simulink model "stateSpace"  (R2023b)
settings: Solver=VariableStepAuto  StartTime=0.0  StopTime=10  RelTol=1e-3  EnableMultiTasking=on
values from neighbouring files (symbols this model uses):
  g = 9.80665    [RegulatorLiniarizare2.m]
  I_r_A = I_r_B + m_r*l_AB^2    (= 0.00169018666667)    [RegulatorLiniarizare2.m]
  I_w_A = I_w_C + m_w*l_AC^2    (= 0.001261425)    [RegulatorLiniarizare2.m]
  I_w_C = 0.5*m_w*R^2    (= 8.6875e-05)    [RegulatorLiniarizare2.m]
  l_AB = l/2    (= 0.065)    [RegulatorLiniarizare2.m]
  l_AC = l    (= 0.13)    [RegulatorLiniarizare2.m]
  m_r = 0.2948    [RegulatorLiniarizare2.m]
  m_w = 0.0695    [RegulatorLiniarizare2.m]
settings Model: Creator=bkhusain  LastModifiedBy=tudorn
settings SolverCC: AlgebraicLoopSolver=TrustRegion
settings DataIOCC: LimitDataPoints=on  MaxDataPoints=10000
settings OptimizationCC: ReuseModelBlockBuffer=off  LifeSpan=inf
settings DebuggingCC: UnconnectedInputMsg=warning  UnconnectedOutputMsg=warning  UnconnectedLineMsg=warning  AllowSymbolicDim=off  SFUnexpectedBacktrackingDiag=warning  SFNoUnconditionalDefaultTransitionDiag=warning  SFExecutionAtInitializationDiag=none  ArithmeticOperatorsInVariantConditions=warning
settings ModelReferenceCC: EnableRefExpFcnMdlSchedulingChecks=on
settings SFSimCC: SimUseLocalCustomCode=off  CustomCodeUndefinedFunction=UseInterfaceOnly
settings RTWCC: RTWUseLocalCustomCode=off
settings CodeAppCC: StateflowObjectComments=on
settings GRTTargetCC: TargetLangStandard=C89/C90 (ANSI)
settings ConfigComp: CovMetricSettings=dw  CovSaveCumulativeToWorkspaceVar=on  CovSaveSingleToWorkspaceVar=on  CovExternalEMLEnable=off  CovSFcnEnable=off
settings SimscapeCC: SimscapeLogType=all  SimscapeLogSimulationStatistics=on  SimscapeLogDataHistory=10000

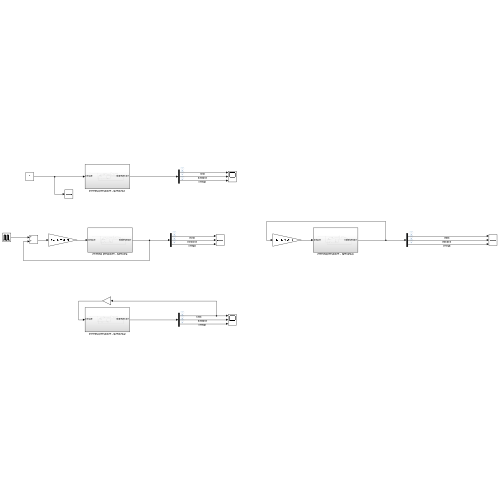
[thumbnail: Simulink's stored preview of the top-level diagram]
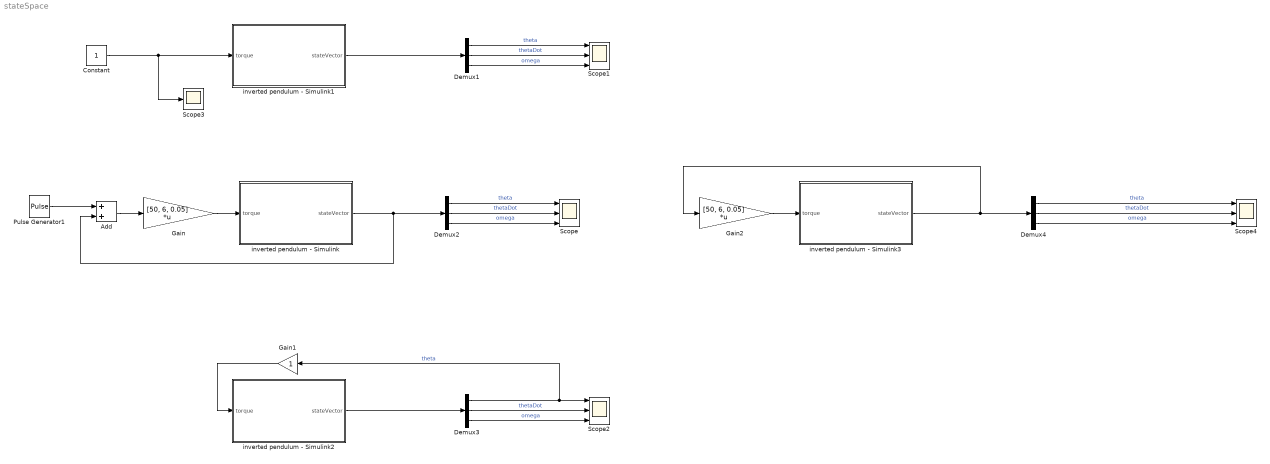
== system stateSpace ==
  Add : Sum
  Constant : Constant
  Demux{1..4} (4 alike) : Demux  Outputs=3
  Gain : Gain  Gain="[50,  6,  0.05]"  Multiplication=Matrix(K*u)
  Gain1 : Gain
  Gain2 : Gain  Gain="[50,  6,  0.05]"  Multiplication=Matrix(K*u)
  Pulse Generator1 : DiscretePulseGenerator  PulseType=Time based  Amplitude=0.5  Period=5  PulseWidth=5
  Scope{,1..2,4} (4 alike) : Scope  NumInputPorts=3
  Scope3 : Scope
  inverted pendulum - Simulink : Subsystem
  inverted pendulum - Simulink1 : Subsystem
  inverted pendulum - Simulink2 : Subsystem
  inverted pendulum - Simulink3 : Subsystem
  wires:
  Demux2/1 -> Scope/1  "theta"
  Demux2/3 -> Scope/3  "omega"
  Demux2/2 -> Scope/2  "thetaDot"
  Gain/1 -> inverted pendulum - Simulink/1(torque)
  Demux1/2 -> Scope1/2  "thetaDot"
  Demux1/3 -> Scope1/3  "omega"
  inverted pendulum - Simulink1/1(stateVector) -> Demux1/1
  Demux1/1 -> Scope1/1  "theta"
  Constant/1 -> Scope3/1, inverted pendulum - Simulink1/1(torque)
  Demux3/2 -> Scope2/2  "thetaDot"
  inverted pendulum - Simulink2/1(stateVector) -> Demux3/1
  Demux3/3 -> Scope2/3  "omega"
  Demux3/1 -> Gain1/1, Scope2/1  "theta"
  Gain1/1 -> inverted pendulum - Simulink2/1(torque)
  Add/1 -> Gain/1
  Pulse Generator1/1 -> Add/1
  inverted pendulum - Simulink/1(stateVector) -> Add/2, Demux2/1
  inverted pendulum - Simulink3/1(stateVector) -> Gain2/1, Demux4/1
  Gain2/1 -> inverted pendulum - Simulink3/1(torque)
  Demux4/2 -> Scope4/2  "thetaDot"
  Demux4/1 -> Scope4/1  "theta"
  Demux4/3 -> Scope4/3  "omega"

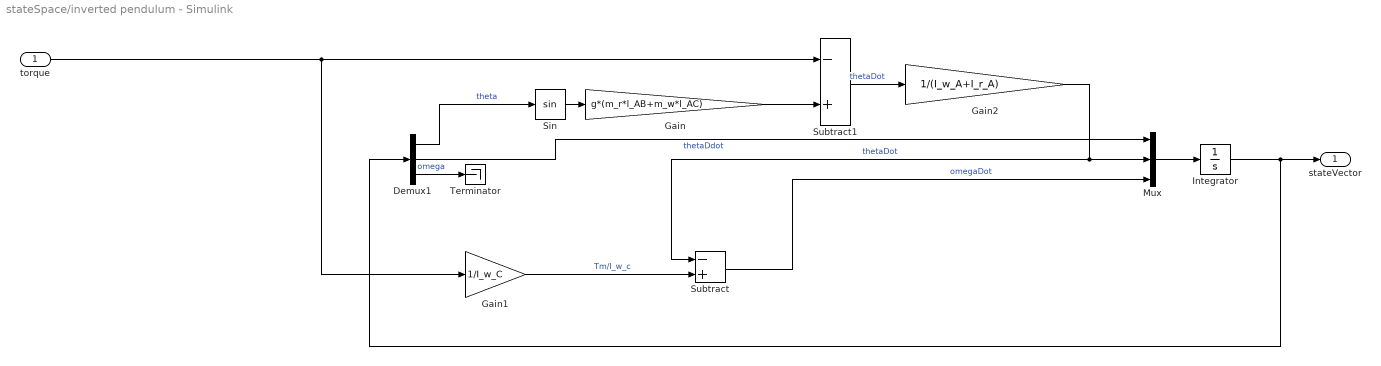
== system stateSpace/inverted pendulum - Simulink ==
  torque : Inport
  Demux1 : Demux  Outputs=3
  Gain : Gain  Gain=g*(m_r*l_AB+m_w*l_AC)
  Gain1 : Gain  Gain=1/I_w_C
  Gain2 : Gain  Gain=1/(I_w_A+I_r_A)
  Integrator : Integrator  InitialCondition=[60*pi/180, 0,0]
  Mux : Mux  Inputs=3
  Sin : Trigonometry
  Subtract : Sum  Inputs=-+
  Subtract1 : Sum  Inputs=-+
  Terminator : Terminator
  stateVector : Outport
  wires:
  Demux1/3 -> Terminator/1  "omega"
  Gain1/1 -> Subtract/2  "Tm/I_w_c"
  Demux1/1 -> Sin/1  "theta"
  Gain2/1 -> Subtract/1, Mux/2  "thetaDot"
  Gain/1 -> Subtract1/2
  Subtract1/1 -> Gain2/1  "thetaDot"
  Subtract/1 -> Mux/3  "omegaDot"
  Demux1/2 -> Mux/1  "thetaDdot"
  torque/1 -> Subtract1/1, Gain1/1
  Sin/1 -> Gain/1
  Integrator/1 -> stateVector/1, Demux1/1
  Mux/1 -> Integrator/1

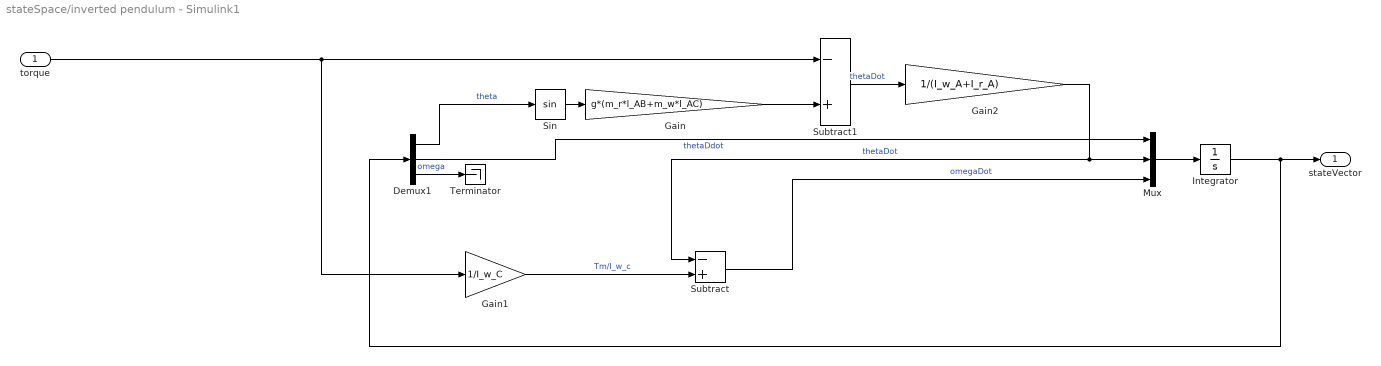
== system stateSpace/inverted pendulum - Simulink1 ==
  torque : Inport
  Demux1 : Demux  Outputs=3
  Gain : Gain  Gain=g*(m_r*l_AB+m_w*l_AC)
  Gain1 : Gain  Gain=1/I_w_C
  Gain2 : Gain  Gain=1/(I_w_A+I_r_A)
  Integrator : Integrator  InitialCondition=[30*pi/180, 0,0]
  Mux : Mux  Inputs=3
  Sin : Trigonometry
  Subtract : Sum  Inputs=-+
  Subtract1 : Sum  Inputs=-+
  Terminator : Terminator
  stateVector : Outport
  wires:
  Demux1/3 -> Terminator/1  "omega"
  Gain1/1 -> Subtract/2  "Tm/I_w_c"
  Demux1/1 -> Sin/1  "theta"
  Gain2/1 -> Subtract/1, Mux/2  "thetaDot"
  Gain/1 -> Subtract1/2
  Subtract1/1 -> Gain2/1  "thetaDot"
  Subtract/1 -> Mux/3  "omegaDot"
  Demux1/2 -> Mux/1  "thetaDdot"
  torque/1 -> Subtract1/1, Gain1/1
  Sin/1 -> Gain/1
  Integrator/1 -> stateVector/1, Demux1/1
  Mux/1 -> Integrator/1

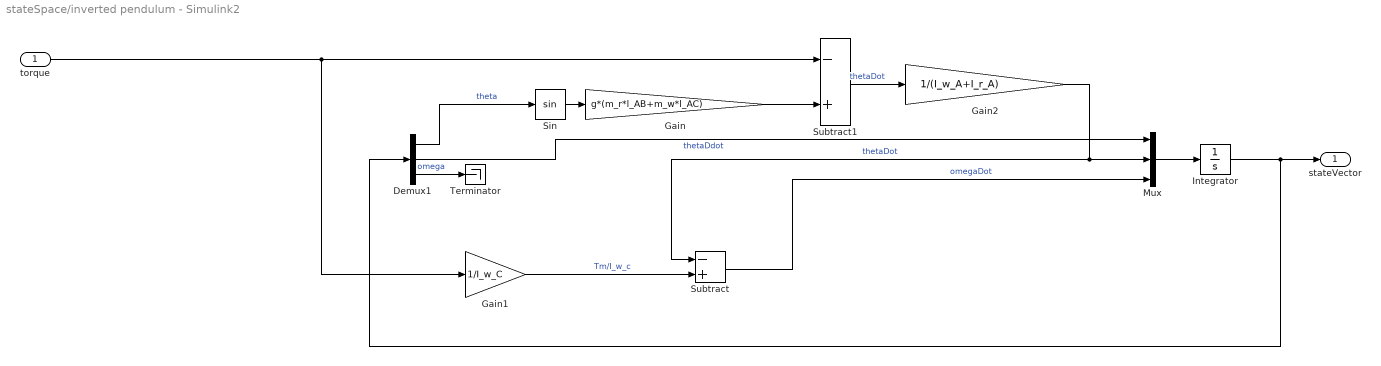
== system stateSpace/inverted pendulum - Simulink2 ==
  torque : Inport
  Demux1 : Demux  Outputs=3
  Gain : Gain  Gain=g*(m_r*l_AB+m_w*l_AC)
  Gain1 : Gain  Gain=1/I_w_C
  Gain2 : Gain  Gain=1/(I_w_A+I_r_A)
  Integrator : Integrator  InitialCondition=[60*pi/180, 0,0]
  Mux : Mux  Inputs=3
  Sin : Trigonometry
  Subtract : Sum  Inputs=-+
  Subtract1 : Sum  Inputs=-+
  Terminator : Terminator
  stateVector : Outport
  wires:
  Demux1/3 -> Terminator/1  "omega"
  Gain1/1 -> Subtract/2  "Tm/I_w_c"
  Demux1/1 -> Sin/1  "theta"
  Gain2/1 -> Subtract/1, Mux/2  "thetaDot"
  Gain/1 -> Subtract1/2
  Subtract1/1 -> Gain2/1  "thetaDot"
  Subtract/1 -> Mux/3  "omegaDot"
  Demux1/2 -> Mux/1  "thetaDdot"
  torque/1 -> Subtract1/1, Gain1/1
  Sin/1 -> Gain/1
  Integrator/1 -> stateVector/1, Demux1/1
  Mux/1 -> Integrator/1

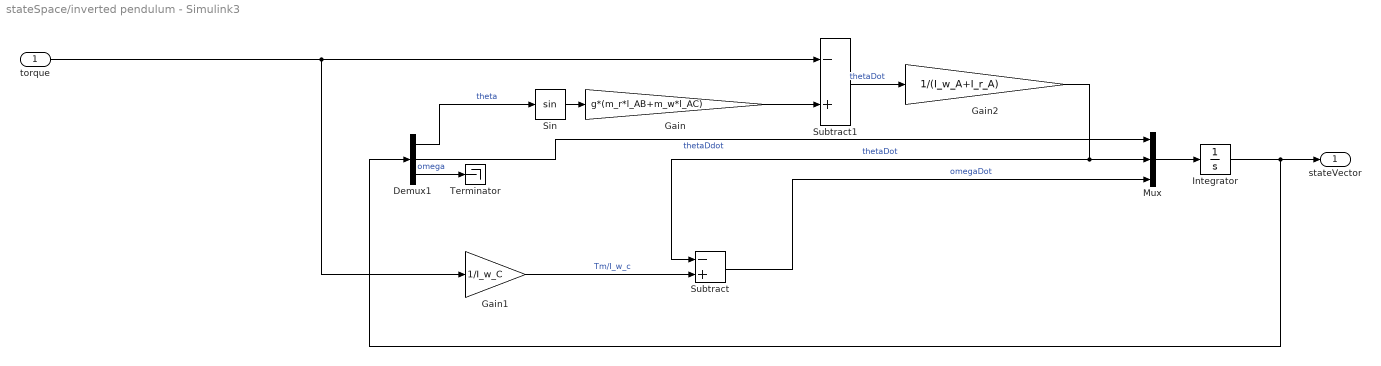
== system stateSpace/inverted pendulum - Simulink3 ==
  torque : Inport
  Demux1 : Demux  Outputs=3
  Gain : Gain  Gain=g*(m_r*l_AB+m_w*l_AC)
  Gain1 : Gain  Gain=1/I_w_C
  Gain2 : Gain  Gain=1/(I_w_A+I_r_A)
  Integrator : Integrator  InitialCondition=[60*pi/180, 0,0]
  Mux : Mux  Inputs=3
  Sin : Trigonometry
  Subtract : Sum  Inputs=-+
  Subtract1 : Sum  Inputs=-+
  Terminator : Terminator
  stateVector : Outport
  wires:
  Demux1/3 -> Terminator/1  "omega"
  Gain1/1 -> Subtract/2  "Tm/I_w_c"
  Demux1/1 -> Sin/1  "theta"
  Gain2/1 -> Subtract/1, Mux/2  "thetaDot"
  Gain/1 -> Subtract1/2
  Subtract1/1 -> Gain2/1  "thetaDot"
  Subtract/1 -> Mux/3  "omegaDot"
  Demux1/2 -> Mux/1  "thetaDdot"
  torque/1 -> Subtract1/1, Gain1/1
  Sin/1 -> Gain/1
  Integrator/1 -> stateVector/1, Demux1/1
  Mux/1 -> Integrator/1
